simulink subsystem "s2e22s"  (R2022b)
settings: Solver=VariableStepAuto  StartTime=0.0  StopTime=10.0  RelTol=1e-3
settings Model: Creator=jack  LastModifiedBy=jack

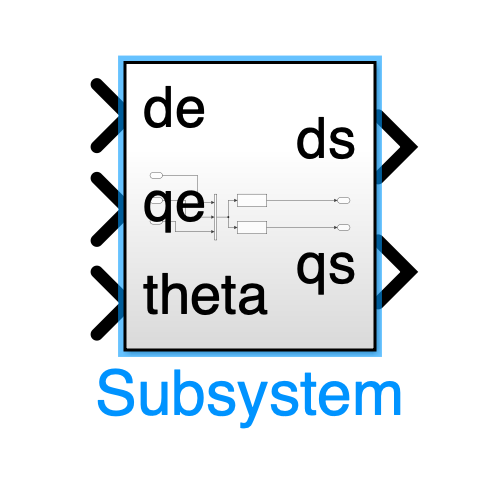
[thumbnail: Simulink's stored preview of the top-level diagram]
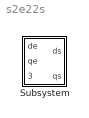
== system s2e22s ==
  Subsystem : Subsystem

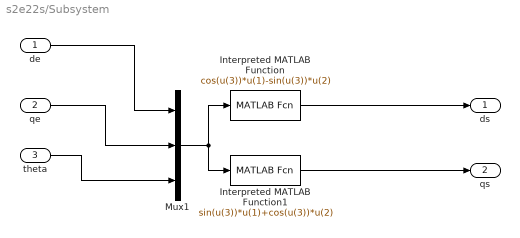
== system s2e22s/Subsystem ==
  de : Inport
  qe : Inport  Port=2
  theta : Inport  Port=3
  Interpreted MATLAB Function : MATLABFcn  MATLABFcn=cos(u(3))*u(1)-sin(u(3))*u(2)
  Interpreted MATLAB Function1 : MATLABFcn  MATLABFcn=sin(u(3))*u(1)+cos(u(3))*u(2)
  Mux1 : Mux  Inputs=3
  ds : Outport
  qs : Outport  Port=2
  wires:
  theta/1 -> Mux1/3
  Interpreted MATLAB Function/1 -> ds/1
  qe/1 -> Mux1/2
  de/1 -> Mux1/1
  Interpreted MATLAB Function1/1 -> qs/1
  Mux1/1 -> Interpreted MATLAB Function/1, Interpreted MATLAB Function1/1
